simulink model "UNIFIER_3DOFsim"  (R2023b)
settings: Solver=VariableStepAuto  StartTime=0  StopTime=t_sim  RelTol=1e-3
InitFcn:
  | UNIFIER_3DOFsim_init
values from neighbouring files (symbols this model uses):
  b = 20.11467    [UNIFIER_LOAD.m]    (also in UNIFIER_LOAD.mat; UNIFIER_LOAD_ROM.m; UNIFIER_LOAD_ROM.mat)
  c = 1.43676    [UNIFIER_LOAD.m]    (also in UNIFIER_LOAD.mat; UNIFIER_LOAD_ROM.m; UNIFIER_LOAD_ROM.mat)
  DEP_inc = -0.0872664625997    [UNIFIER_LOAD.mat]    (also in UNIFIER_ROMdyn.m = deg2rad(-5); UNIFIER_ROMdyn_script.m = deg2rad(-5); UNIFIER_ROMdyn_v2.m = deg2rad(-5); UNIFIER_ROMgen.m = 0.1)
  dp_DEP =     [UNIFIER_LOAD.mat]    (also in UNIFIER_LOAD_ROM.mat)
  dp_FUSE_FIN =     [UNIFIER_LOAD.mat]
  dp_HTU =     [UNIFIER_LOAD.mat]    (also in UNIFIER_LOAD_ROM.mat)
  dp_VTAIL =     [UNIFIER_LOAD.mat]
  dp_VTAIL_INDUCED =     [UNIFIER_LOAD.mat]
  dp_WING_root =     [UNIFIER_LOAD.mat]
  dp_WING_tip =     [UNIFIER_LOAD.mat]
  dumax = [2.09439510239 2.09439510239 2.09439510239 1.0471975512 2 4 2]    [UNIFIER_LOAD.mat]    (also in UNIFIER_LOAD_ROM.mat = [1.0471975512 1.0471975512 1.0471975512 0.174532925199 2 2 2)
  gr = 9.80665    [UNIFIER_LOAD.mat]    (also in UNIFIER_LOAD_ROM.mat)
  m = 7057    [UNIFIER_LOAD.m]    (also in UNIFIER_LOAD.mat; UNIFIER_LOAD_ROM.m; UNIFIER_LOAD_ROM.mat)
  n_prop = 12    [UNIFIER_LOAD.mat]    (also in UNIFIER_ROMdyn.m; UNIFIER_ROMdyn_script.m; UNIFIER_ROMdyn_v2.m)
  prop_d = 1.6    [UNIFIER_LOAD.mat]    (also in UNIFIER_ROMdyn.m; UNIFIER_ROMdyn_script.m; UNIFIER_ROMdyn_v2.m)
  ROMv1 = ROM    [UNIFIER_3DOFsim_init.m]    (also in UNIFIER_ROMgen_subset.m; UNIFIER_ROMgen_v2_subset.m; UNIFIER_ROMgen_v3_subset.m; UNIFIER_ROMgen_v4_subset.m)
  ROMv2 = ROM    [UNIFIER_3DOFsim_init.m]
  ROMv3 = ROM    [UNIFIER_3DOFsim_init.m]
  S = 29.98388    [UNIFIER_LOAD.m]    (also in UNIFIER_LOAD.mat; UNIFIER_LOAD_ROM.m; UNIFIER_LOAD_ROM.mat)
  U_trim = [ustar(3) ... (first row only)    [UNIFIER_3DOFsim_init.m]
  umax = inf    [UNIFIERLanding.m]    (also in UNIFIER_LOAD.mat = [0.436332312999 0.523598775598 0.523598775598 0.436332312999; UNIFIER_LOAD_ROM.mat = [0.436332312999 0.523598775598 0.349065850399 0.436332312999)
  umin = 0    [UNIFIERLanding.m]    (also in UNIFIER_LOAD.mat = [-0.436332312999 -0.523598775598 -0.523598775598 0 0 -1 -0.5; UNIFIER_LOAD_ROM.mat = [-0.436332312999 -0.523598775598 -0.0872664625997 0 0 -1 0])
  Va = sqrt(u^2+w^2)    [ROMcomp.m]    (also in UNIFIERLanding.m = sqrt(x(:,3).^2+x(:,4).^2); UNIFIERLanding_Dynamics_Internal.m = sqrt(X(:,3).^2+X(:,4).^2); UNIFIERLanding_Main.m = sqrt(solution.X(:,3).^2+solution.X(:,4).^2); UNIFIERLanding_trajopt.m = sqrt(solution.X(:,3).^2+solution.X(:,4).^2))
  vtail_nodes = [dp_VTAIL.Xs_LE;     dp_VTAIL.Ys_LE;     dp_VTAIL.Zs_LE]    [UNIFIER_LOAD.m]    (also in UNIFIER_LOAD.mat = [-16.4894695282 -2.83441376686 -2.73765826225 -16.1370849609)
  wing_nodes = [fliplr(dp_WING_tip.LE_Xs),fliplr(dp_WING_root.LE_Xs),dp_WING_root.LE_Xs,dp_WING_tip.LE_Xs;     fliplr(-dp_WING_tip.LE_Ys),fliplr(-dp_WING_root.LE_Ys),dp_WING_root.LE_Ys,dp_WING_tip.LE_Ys;     fliplr(dp_WING_tip.LE_Zs),fliplr(dp_WING_root.LE_Zs),dp_WING_root.LE_Zs,dp_WING_tip.LE_Zs]    [UNIFIER_LOAD.m]    (also in UNIFIER_LOAD.mat = [-7.70795631409 -9.67500019073 -0.98178178072 -7.66801691055)
  x0 = xstar(1)    [UNIFIERLanding.m]    (also in UNIFIER_3DOFsim_init.m; UNIFIER_dynamics.m = x; UNIFIER_trim.m = [Va_target/100; UNIFIER_trim1.m = [Va_target)
  xstar = [0;        0;        -ze_target;        zstar(1)*100;        0;        zstar(2)*100;        0;        zstar(3);        0;        0;        0;        0]    [UNIFIER_trim.m]    (also in UNIFIER_trim0_res.mat = [0 0 -500 55.1327882403 0 -0.446351795968 0 1.36591182427e-0; UNIFIER_trim1.m = [0;        0;        -ze_target;        zstar(1);        0; ; UNIFIER_trim1_res.mat = [0 0 -1219 72.7310470326 0 1.14230710452 0 0.0157060522827 0; UNIFIER_trimHFM.m = [0;        0;        -runconfig.ze;        zstar(1)*100;    )
  xyz_cg = [-8.09,0,-0.2]    [UNIFIER_LOAD.m]    (also in UNIFIER_LOAD.mat = [-8.09 0 -0.2]; UNIFIER_LOAD_ROM.m; UNIFIER_LOAD_ROM.mat = [-8.09 0 -0.2])
  xyz_cg_12 = [-8.09 0 -0.2 -8.09 0 -0.2 -8.09 0 -0.2 -8.09 0 -0.2 ... (36 elements, 3x12)]    [UNIFIER_LOAD.mat]    (also in UNIFIER_LOAD_ROM.mat)
  xyz_DEP = [ -6.9629998	-6.9210000	-6.8660002	-6.8099999	-6.7540002	-6.6999998	-6.6999998	-6.7540002	-6.8099999	-6.8660002	-6.9210000	-6.9629998 ... (first row only)    [UNIFIER_LOAD.m]    (also in UNIFIER_LOAD.mat = [-6.9629998 -10.05 -0.90899998 -6.921 -8.4499998 -0.792 -6.8; UNIFIER_LOAD_ROM.m; UNIFIER_LOAD_ROM.mat = [-6.9629998 -10.05 -0.90899998 -6.921 -8.4499998 -0.792 -6.8)
  z0 = x(1,2)    [UNIFIERLanding.m]    (also in UNIFIER_3DOFsim_init.m = xstar(3); UNIFIER_trim.m = zstar; UNIFIER_trim1.m = zstar; UNIFIER_trimHFM.m = zstar)
undefined symbols (not defined in the file or in its folder): solution
libraries: simulink_extras x17, sharedutil x5, slpidlib x4, aerolibtransform2 x4, dspindex x2, matrix_library x1, shared6dof x1, aerolibatmos2 x1, simulink x1
(part 1 of 4)
settings Model: Creator=Reggie Johanes  LastModifiedBy=Reggie Johanes
settings DataIOCC: SaveFormat=StructureWithTime
settings OptimizationCC: BlockReduction=off  BufferReuse=off
settings DebuggingCC: AlgebraicLoopMsg=none  ParameterPrecisionLossMsg=none

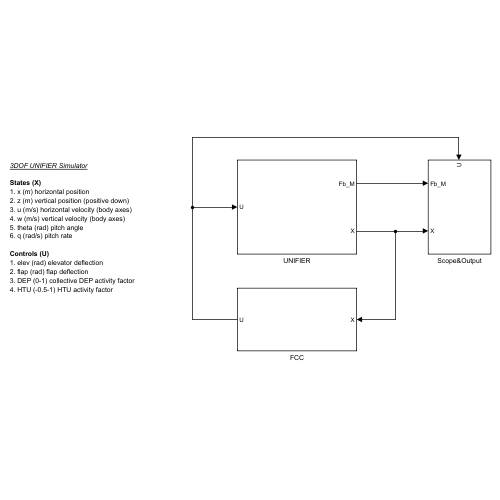
[thumbnail: Simulink's stored preview of the top-level diagram]
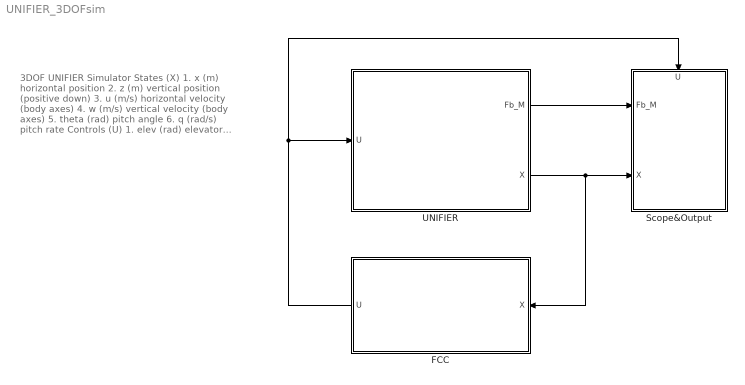
== system UNIFIER_3DOFsim ==
  note: 3DOF UNIFIER Simulator
      |
      | States (X)
      | 1. x (m) horizontal position
      | 2. z (m) vertical position (positive down)
      | 3. u (m/s) horizontal velocity (body axes)
      | 4. w (m/s) vertical velocity (body axes)
      | 5. theta (rad) pitch angle
      | 6. q (rad/s) pitch rate
      |
      | Controls (U)
      | 1. elev (rad) elevator deflection
      | 2. flap (rad) flap deflection
      | 3. DEP (0-1) collective DEP activity factor
      | 4. HTU (-0.5-1) HTU activity factor
  FCC : Subsystem
  Scope&Output : Subsystem
      settings: PortSchema="{\"entries\":[{\"content\":{\"sides\":[{\"content\":{\"connectorIds\":[\"In1\",\"In2\"]},\"type\":\"ConnectorPlacement.EquallySpacedRectSide\",\"uuid\":\"009958d8-f299-4591-8265-ecda8c772736\"},{\"content\":{\"side\":\"RIGHT\"},\"type\":\"ConnectorPlacement.EquallySpacedRectSide\",\"uuid\":\"c33e155a-8705-44ed-ad70-cac76bf4a7ef\"},{\"content\":{\"connectorIds\":[\"In3\"],\"side\":\"TOP\"},\"type\":\"ConnectorPlacement.EquallySpacedRectSide\",\"uuid\":\"edbc7869-8e0d-4a22-bba1-11cba2971ecb\"}]},\"type\":\"ConnectorPlacement.EquallySpacedConnector\",\"uuid\":\"bd1ea077-c17e-402d-9949-f0df00fcfe32\"}],\"packageUris\":[\"http://schema.mathworks.com/mf0/Connector/R2020b\"],\"version\":\"1.0\"}"
  UNIFIER : Subsystem
  wires:
  UNIFIER/2(X) -> FCC/1(X), Scope&Output/2(X)
  FCC/1(U) -> UNIFIER/1(U), Scope&Output/3(U)
  UNIFIER/1(Fb_M) -> Scope&Output/1(Fb_M)

== system UNIFIER_3DOFsim/FCC ==
  X : Inport
  Airspeed Control : Subsystem
      settings: PortSchema="{\"entries\":[{\"content\":{\"sides\":[{\"content\":{\"connectorIds\":[\"In1\",\"In2\"]},\"type\":\"ConnectorPlacement.EquallySpacedRectSide\",\"uuid\":\"a3fb04a8-89c2-4134-89d4-6d6a43062b9b\"},{\"content\":{\"connectorIds\":[\"Out1\"],\"side\":\"RIGHT\"},\"type\":\"ConnectorPlacement.EquallySpacedRectSide\",\"uuid\":\"0d35a5ec-1bbb-45b5-ad25-2bc644cb46ec\"},{\"content\":{\"connectorIds\":[\"Out2\"],\"side\":\"TOP\"},\"type\":\"ConnectorPlacement.EquallySpacedRectSide\",\"uuid\":\"07800402-c5fd-46cf-bb6b-6507cb62190b\"}]},\"type\":\"ConnectorPlacement.EquallySpacedConnector\",\"uuid\":\"0f781fd0-6236-48b8-b612-1777b9bca292\"}],\"packageUris\":[\"http://schema.mathworks.com/mf0/Connector/R2020b\"],\"version\":\"1.0\"}"
  Altitude Control : Subsystem
      settings: PortSchema="{\"entries\":[{\"content\":{\"sides\":[{\"content\":{\"connectorIds\":[\"In1\",\"In2\",\"In3\",\"In4\"]},\"type\":\"ConnectorPlacement.EquallySpacedRectSide\",\"uuid\":\"d6eebd62-3574-4a6b-be51-6258a51c0c28\"},{\"content\":{\"connectorIds\":[\"Out1\"],\"side\":\"RIGHT\"},\"type\":\"ConnectorPlacement.EquallySpacedRectSide\",\"uuid\":\"54870a02-b95d-471b-a2c8-ee83b599c45e\"},{\"content\":{\"side\":\"TOP\"},\"type\":\"ConnectorPlacement.EquallySpacedRectSide\",\"uuid\":\"efdc830e-c8bf-412c-9d86-dbb1e6c1c86b\"},{\"content\":{\"connectorIds\":[\"Out2\"],\"side\":\"BOTTOM\"},\"type\":\"ConnectorPlacement.EquallySpacedRectSide\",\"uuid\":\"beb3ac17-a4c7-4320-a029-baa0478db22b\"}]},\"type\":\"ConnectorPlacement.EquallySpacedConnector\",\"uuid\":\"0f69f6a5-bc47-4551-ad8e-935190b4abb2\"}],\"packageUris\":[\"http://schema.mathworks.com/mf0/Connector/R2020b\"],\"version\":\"1.0\"}"
  Bus Selector : BusSelector  OutputSignals=Va_tas,xe,ze,theta,q
  Constant : Constant  Value=U_trim
  Demux : Demux
  From : From
  Gain : Gain  Commented=through  Gain=0
  Gain1 : Gain  Commented=through  Gain=0
  Goto : Goto
  Mux : Mux
  Sat&RateLimits : Subsystem
  Scopes : Subsystem
      settings: PortSchema="{\"entries\":[{\"content\":{\"sides\":[{\"content\":{},\"type\":\"ConnectorPlacement.EquallySpacedRectSide\",\"uuid\":\"9f44d661-c392-453f-8f32-a438acdd3e9a\"},{\"content\":{\"connectorIds\":[\"In1\",\"In2\",\"In3\",\"In4\"],\"side\":\"RIGHT\"},\"type\":\"ConnectorPlacement.EquallySpacedRectSide\",\"uuid\":\"1fec26d2-6697-4a56-8467-3c40b28ed85c\"},{\"content\":{\"side\":\"TOP\"},\"type\":\"ConnectorPlacement.EquallySpacedRectSide\",\"uuid\":\"ddff103d-3713-4047-b105-bfe64402e206\"}]},\"type\":\"ConnectorPlacement.EquallySpacedConnector\",\"uuid\":\"f87a61e9-3668-4a68-bbee-b53c56c665da\"}],\"packageUris\":[\"http://schema.mathworks.com/mf0/Connector/R2020b\"],\"version\":\"1.0\"}"
  Sum : Sum  Inputs=|++
  Sum1 : Sum  Inputs=|++
  Sum2 : Sum  Inputs=|++
  U : Outport
  wires:
  X/1 -> [C], Bus Selector/1
  Constant/1 -> Demux/1
  Sat&RateLimits/1(U_lim) -> U/1, Scopes/4(U)
  Mux/1 -> Sat&RateLimits/1(U)
  Sum/1 -> Mux/1  "elev"
  Demux/1 -> Sum/2
  Demux/3 -> Sum1/2
  Demux/4 -> Sum2/2
  Sum2/1 -> Mux/4  "HTU"
  Sum1/1 -> Mux/3  "DEP"
  Demux/2 -> Mux/2  "flap"
  Altitude Control/1(elev) -> Gain/1
  Airspeed Control/1(thr) -> Gain1/1
  Bus Selector/1 -> Airspeed Control/1(Va)  "<Va_tas>"
  Bus Selector/2 -> Airspeed Control/2(Xe), Altitude Control/4(Xe)  "<xe>"
  Bus Selector/3 -> Altitude Control/1(Ze)  "<ze>"
  Bus Selector/4 -> Altitude Control/2(theta)  "<theta>"
  Bus Selector/5 -> Altitude Control/3(q)  "<q>"
  Airspeed Control/2(scopeout) -> Goto/1
  Altitude Control/2(scopeout) -> [B]
  From/1 -> Scopes/1(Vactrl)
  [B] -> Scopes/2(altctrl)
  [C] -> Scopes/3(X)
  Gain/1 -> Sum/1
  Gain1/1 -> Sum2/1, Sum1/1

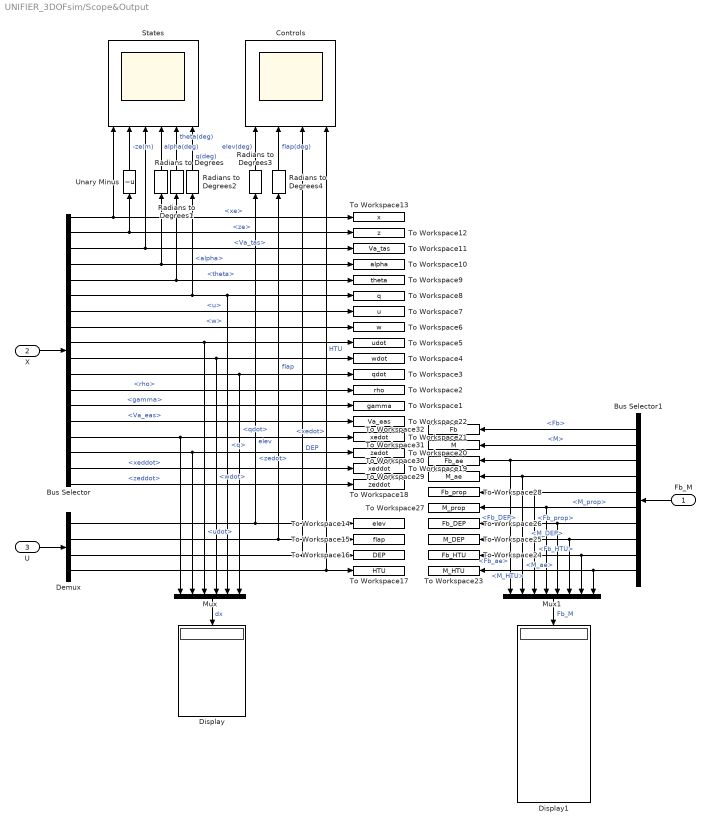
== system UNIFIER_3DOFsim/Scope&Output ==
  Fb_M : Inport
  X : Inport  Port=2
  U : Inport  Port=3
  Bus Selector : BusSelector  OutputSignals=xe,ze,Va_tas,alpha,theta,q,u,w,udot,wdot,qdot,rho,gamma,Va_eas,xedot,zedot,xeddot,zeddot
  Bus Selector1 : BusSelector  OutputSignals=Fb,M,Fb_ae,M_ae,Fb_prop,M_prop,Fb_DEP,M_DEP,Fb_HTU,M_HTU
  Controls : Scope  NumInputPorts=4
  Demux : Demux
  Display : Display
  Display1 : Display
  Mux : Mux  Inputs=6
  Mux1 : Mux  Inputs=8
  Radians to Degrees{,1..4} (5 alike) : simulink_extras/Transformations/Radians to Degrees
  States : Scope  NumInputPorts=6
  To Workspace1 : ToWorkspace  VariableName=gamma  SampleTime=-1
  To Workspace10 : ToWorkspace  VariableName=alpha  SampleTime=-1
  To Workspace11 : ToWorkspace  VariableName=Va_tas  SampleTime=-1
  To Workspace12 : ToWorkspace  VariableName=z  SampleTime=-1
  To Workspace13 : ToWorkspace  VariableName=x  SampleTime=-1
  To Workspace14 : ToWorkspace  VariableName=elev  SampleTime=-1
  To Workspace15 : ToWorkspace  VariableName=flap  SampleTime=-1
  To Workspace16 : ToWorkspace  VariableName=DEP  SampleTime=-1
  To Workspace17 : ToWorkspace  VariableName=HTU  SampleTime=-1
  To Workspace18 : ToWorkspace  VariableName=zeddot  SampleTime=-1
  To Workspace19 : ToWorkspace  VariableName=xeddot  SampleTime=-1
  To Workspace2 : ToWorkspace  VariableName=rho  SampleTime=-1
  To Workspace20 : ToWorkspace  VariableName=zedot  SampleTime=-1
  To Workspace21 : ToWorkspace  VariableName=xedot  SampleTime=-1
  To Workspace22 : ToWorkspace  VariableName=Va_eas  SampleTime=-1
  To Workspace23 : ToWorkspace  VariableName=M_HTU  SampleTime=-1
  To Workspace24 : ToWorkspace  VariableName=Fb_HTU  SampleTime=-1
  To Workspace25 : ToWorkspace  VariableName=M_DEP  SampleTime=-1
  To Workspace26 : ToWorkspace  VariableName=Fb_DEP  SampleTime=-1
  To Workspace27 : ToWorkspace  VariableName=M_prop  SampleTime=-1
  To Workspace28 : ToWorkspace  VariableName=Fb_prop  SampleTime=-1
  To Workspace29 : ToWorkspace  VariableName=M_ae  SampleTime=-1
  To Workspace3 : ToWorkspace  VariableName=qdot  SampleTime=-1
  To Workspace30 : ToWorkspace  VariableName=Fb_ae  SampleTime=-1
  To Workspace31 : ToWorkspace  VariableName=M  SampleTime=-1
  To Workspace32 : ToWorkspace  VariableName=Fb  SampleTime=-1
  To Workspace4 : ToWorkspace  VariableName=wdot  SampleTime=-1
  To Workspace5 : ToWorkspace  VariableName=udot  SampleTime=-1
  To Workspace6 : ToWorkspace  VariableName=w  SampleTime=-1
  To Workspace7 : ToWorkspace  VariableName=u  SampleTime=-1
  To Workspace8 : ToWorkspace  VariableName=q  SampleTime=-1
  To Workspace9 : ToWorkspace  VariableName=theta  SampleTime=-1
  Unary Minus : UnaryMinus
  wires:
  X/1 -> Bus Selector/1
  Bus Selector/1 -> States/1, To Workspace13/1  "<xe>"
  Bus Selector/2 -> Unary Minus/1, To Workspace12/1  "<ze>"
  Bus Selector/3 -> States/3, To Workspace11/1  "<Va_tas>"
  Bus Selector/4 -> Radians to Degrees/1, To Workspace10/1  "<alpha>"
  Bus Selector/5 -> Radians to Degrees1/1, To Workspace9/1  "<theta>"
  Bus Selector/6 -> Radians to Degrees2/1, To Workspace8/1, Mux/5  "<q>"
  Bus Selector/8 -> To Workspace6/1  "<w>"
  Bus Selector/9 -> To Workspace5/1, Mux/3  "<udot>"
  Bus Selector/10 -> To Workspace4/1, Mux/4  "<wdot>"
  Bus Selector/11 -> To Workspace3/1, Mux/6  "<qdot>"
  Bus Selector/12 -> To Workspace2/1  "<rho>"
  Bus Selector/13 -> To Workspace1/1  "<gamma>"
  Bus Selector/7 -> To Workspace7/1  "<u>"
  U/1 -> Demux/1
  Demux/1 -> Radians to Degrees3/1, To Workspace14/1  "elev"
  Demux/2 -> To Workspace15/1, Radians to Degrees4/1  "flap"
  Demux/3 -> To Workspace16/1, Controls/3  "DEP"
  Demux/4 -> To Workspace17/1, Controls/4  "HTU"
  Radians to Degrees/1 -> States/4  "alpha(deg)"
  Radians to Degrees1/1 -> States/5  "theta(deg)"
  Radians to Degrees2/1 -> States/6  "q(deg)"
  Radians to Degrees3/1 -> Controls/1  "elev(deg)"
  Radians to Degrees4/1 -> Controls/2  "flap(deg)"
  Unary Minus/1 -> States/2  "-ze(m)"
  Bus Selector/14 -> To Workspace22/1  "<Va_eas>"
  Bus Selector/15 -> To Workspace21/1, Mux/1  "<xedot>"
  Bus Selector/16 -> To Workspace20/1, Mux/2  "<zedot>"
  Bus Selector/17 -> To Workspace19/1  "<xeddot>"
  Bus Selector/18 -> To Workspace18/1  "<zeddot>"
  Mux/1 -> Display/1  "dx"
  Fb_M/1 -> Bus Selector1/1
  Bus Selector1/3 -> To Workspace30/1, Mux1/1  "<Fb_ae>"
  Bus Selector1/4 -> To Workspace29/1, Mux1/2  "<M_ae>"
  Bus Selector1/5 -> To Workspace28/1, Mux1/3  "<Fb_prop>"
  Bus Selector1/6 -> Mux1/4, To Workspace27/1  "<M_prop>"
  Bus Selector1/7 -> To Workspace26/1, Mux1/5  "<Fb_DEP>"
  Bus Selector1/8 -> To Workspace25/1, Mux1/6  "<M_DEP>"
  Bus Selector1/9 -> To Workspace24/1, Mux1/7  "<Fb_HTU>"
  Bus Selector1/10 -> To Workspace23/1, Mux1/8  "<M_HTU>"
  Mux1/1 -> Display1/1  "Fb_M"
  Bus Selector1/1 -> To Workspace32/1  "<Fb>"
  Bus Selector1/2 -> To Workspace31/1  "<M>"

== system UNIFIER_3DOFsim/UNIFIER ==
  U : Inport
  Aerodynamics : Subsystem
      settings: PortSchema="{\"entries\":[{\"content\":{\"sides\":[{\"content\":{\"connectorIds\":[\"In1\",\"In2\"]},\"type\":\"ConnectorPlacement.EquallySpacedRectSide\",\"uuid\":\"e9d20c59-d6d6-400e-86e2-7a5ce5b582a2\"},{\"content\":{\"connectorIds\":[\"Out1\"],\"side\":\"RIGHT\"},\"type\":\"ConnectorPlacement.EquallySpacedRectSide\",\"uuid\":\"90d146c5-a119-4790-99ca-b691f9272bd7\"},{\"content\":{\"side\":\"TOP\"},\"type\":\"ConnectorPlacement.EquallySpacedRectSide\",\"uuid\":\"d5361e2b-6780-4a80-8d58-884ba2a6b49f\"},{\"content\":{\"connectorIds\":[\"In3\"],\"side\":\"BOTTOM\"},\"type\":\"ConnectorPlacement.EquallySpacedRectSide\",\"uuid\":\"13a1fcba-5f98-490a-a419-e6367cfc3f2c\"}]},\"type\":\"ConnectorPlacement.EquallySpacedConnector\",\"uuid\":\"a6bcc40b-a991-474d-9674-c204f7c17676\"}],\"packageUris\":[\"http://schema.mathworks.com/mf0/Connector/R2020b\"],\"version\":\"1.0\"}"
  EOM&Environment : Subsystem
      settings: PortSchema="{\"entries\":[{\"content\":{\"sides\":[{\"content\":{\"connectorIds\":[\"In1\"]},\"type\":\"ConnectorPlacement.EquallySpacedRectSide\",\"uuid\":\"6160da2b-8552-4ec1-894a-26a5f6c45b78\"},{\"content\":{\"connectorIds\":[\"Out1\",\"Out2\"],\"side\":\"RIGHT\"},\"type\":\"ConnectorPlacement.EquallySpacedRectSide\",\"uuid\":\"7b74025f-6315-4fda-9352-f522b3ee102f\"},{\"content\":{\"side\":\"TOP\"},\"type\":\"ConnectorPlacement.EquallySpacedRectSide\",\"uuid\":\"a0b3834c-0ad6-468f-a161-0f220b7032c2\"},{\"content\":{\"connectorIds\":[\"In2\"],\"side\":\"BOTTOM\"},\"type\":\"ConnectorPlacement.EquallySpacedRectSide\",\"uuid\":\"9d5650a6-6ba4-451c-b870-367e56356c4c\"}]},\"type\":\"ConnectorPlacement.EquallySpacedConnector\",\"uuid\":\"bb7293ac-4d3c-4803-b4ea-767d72af75c5\"}],\"packageUris\":[\"http://schema.mathworks.com/mf0/Connector/R2020b\"],\"version\":\"1.0\"}"
  Propulsion : Subsystem
      settings: PortSchema="{\"entries\":[{\"content\":{\"sides\":[{\"content\":{\"connectorIds\":[\"In1\",\"In2\"]},\"type\":\"ConnectorPlacement.EquallySpacedRectSide\",\"uuid\":\"59a18027-8e03-454d-b478-7172993824c1\"},{\"content\":{\"connectorIds\":[\"Out1\"],\"side\":\"RIGHT\"},\"type\":\"ConnectorPlacement.EquallySpacedRectSide\",\"uuid\":\"f9f30e45-7108-4b05-88e5-0eee1548e389\"},{\"content\":{\"connectorIds\":[\"Out2\"],\"side\":\"TOP\"},\"type\":\"ConnectorPlacement.EquallySpacedRectSide\",\"uuid\":\"8bce0bfc-d093-42df-8b33-22202eb99c5b\"}]},\"type\":\"ConnectorPlacement.EquallySpacedConnector\",\"uuid\":\"2f803787-601f-4bf2-b234-403b5a693950\"}],\"packageUris\":[\"http://schema.mathworks.com/mf0/Connector/R2020b\"],\"version\":\"1.0\"}"
  Fb_M : Outport
  X : Outport  Port=2
  wires:
  Propulsion/1(Fb_M_prop) -> EOM&Environment/2(Fb_M_prop)
  U/1 -> Aerodynamics/2(U), Propulsion/1(U)
  Propulsion/2(J) -> Aerodynamics/3(J)
  Aerodynamics/1(Fb_M_ae) -> EOM&Environment/1(Fb_M_ae)
  EOM&Environment/1(X) -> X/1, Propulsion/2(X), Aerodynamics/1(X)
  EOM&Environment/2(Fb_M) -> Fb_M/1

== system UNIFIER_3DOFsim/FCC/Airspeed Control ==
  Va : Inport
  Xe : Inport  Port=2
  1-D Lookup Table : Lookup_n-D  NumberOfTableDimensions=1  BreakpointsForDimension1=solution.X(:,1)  Table=Va  InternalRulePriority=Speed  RndMeth=Simplest
  1-D Lookup Table1 : Lookup_n-D  Commented=on  NumberOfTableDimensions=1  BreakpointsForDimension1=solution.T  Table=Va  InternalRulePriority=Speed  RndMeth=Simplest
  Bus Creator : BusCreator  Inputs=2
  Clock : Clock  Commented=on
  PID_Va : slpidlib/PID Controller  Controller=PI  Form=Parallel  TimeDomain=Continuous-time  UseExternalTs=off  SampleTime=-1  IntegratorMethod=Forward Euler  FilterMethod=Forward Euler  ControllerParametersSource=internal  P=1.5  I=0.5  UseKiTs=off  D=0.001  N=0  UseFilter=on  TunerSelectOption=Transfer Function Based (PID Tuner App)  InitialConditionSource=internal  InitialConditionForIntegrator=0  InitialConditionForFilter=0  DifferentiatorICPrevScaledInput=0  ExternalReset=none  TrackingMode=off  Kt=1  LimitOutput=off  SatLimitsSource=internal  UpperSaturationLimit=inf  LowerSaturationLimit=-inf  LinearizeAsGain=on  AntiWindupMode=none  Kb=1  LimitIntegrator=off  UpperIntegratorSaturationLimit=inf  LowerIntegratorSaturationLimit=-inf  POutMin=[]  POutMax=[]  IOutMin=[]  IOutMax=[]  DOutMin=[]  DOutMax=[]  NOutMin=[]  NOutMax=[]  SumOutMin=[]  SumOutMax=[]  SaturationOutMin=[]  SaturationOutMax=[]  PParamMin=[]  PParamMax=[]  IParamMin=[]  IParamMax=[]  DParamMin=[]  DParamMax=[]  NParamMin=[]  NParamMax=[]  KbParamMin=[]  KbParamMax=[]  KtParamMin=[]  KtParamMax=[]  KbOutMin=[]  KbOutMax=[]  KtOutMin=[]  KtOutMax=[]  IntegratorOutMin=[]  IntegratorOutMax=[]  FilterOutMin=[]  FilterOutMax=[]  SumI1OutMin=[]  SumI1OutMax=[]  SumI2OutMin=[]  SumI2OutMax=[]  SumI3OutMin=[]  SumI3OutMax=[]  SumI4OutMin=[]  SumI4OutMax=[]  SumDOutMin=[]  SumDOutMax=[]  DifferentiatorOutMin=[]  DifferentiatorOutMax=[]  FilterDiffOutCoefMin=[]  FilterDiffOutCoefMax=[]  ReciprocalOutMin=[]  ReciprocalOutMax=[]  SumDenOutMin=[]  SumDenOutMax=[]  SumNumOutMin=[]  SumNumOutMax=[]  DivideOutMin=[]  DivideOutMax=[]  UdiffTsProdOutMin=[]  UdiffTsProdOutMax=[]  NTsProdOutMin=[]  NTsProdOutMax=[]  UintegralTsProdOutMin=[]  UintegralTsProdOutMax=[]  UngainTsProdOutMin=[]  UngainTsProdOutMax=[]  ClampingZeroOutDataTypeStr=Inherit: Inherit via back propagation  ClampingZeroOutMin=[]  ClampingZeroOutMax=[]  FilterDenConstantOutDataTypeStr=Inherit: Inherit via back propagation  FilterDenConstantOutMin=[]  FilterDenConstantOutMax=[]  PCopyOutDataTypeStr=Inherit: Inherit via back propagation  PCopyOutMin=[]  PCopyOutMax=[]  NCopyOutDataTypeStr=Inherit: Inherit via back propagation  NCopyOutMin=[]  NCopyOutMax=[]  IntegratorContinuousStateAttributes=''  IntegratorStateMustResolveToSignalObject=off  IntegratorRTWStateStorageClass=Auto  FilterContinuousStateAttributes=''  FilterStateMustResolveToSignalObject=off  FilterRTWStateStorageClass=Auto  ParallelPVariant=InternalParameters  IdealPVariant=Disabled  IVariant=InternalParameters  DVariant=Disabled  IntegratorVariant=Continuous  SatVariant=Disabled  AWVariant=Passthrough  PCopyVariant=Disabled  TRVariant=Disabled  FdbkBlocksVariant=Forward  IdealPFdbkVariant=Disabled  SatFdbkVariant=Disabled  DerivativeFilterVariant=Disabled  NVariant=Disabled  NCopyVariant=Disabled_SignalSpec  FilterICVariant=Disabled  IntegratorICVariant=InternalICs  ExternalResetVariant=Disabled  TRSumVariant=Passthrough  SumFdbkVariant=Disabled  SumVariant=Sum_PI  TsampFilterVariant=InternalTs  TsampNgainVariant=Passthrough  TsampIntegralVariant=Disabled_SignalSpec  ExternalSaturationOutDataTypeStr=Inherit: Same as second input
  Sum : Sum  Inputs=|+-
  Sum1 : Sum  Inputs=++|
  Va_ctrl : Scope  NumInputPorts=2
  Va_step : Step  Commented=on  Time=5  Before=72.74  After=72.74  SampleTime=0
  thr : Outport
  scopeout : Outport  Port=2
  wires:
  Va/1 -> Va_ctrl/2, Sum/2
  Sum/1 -> PID_Va/1
  PID_Va/1 -> Bus Creator/2, thr/1  "thr_cmd"
  Xe/1 -> 1-D Lookup Table/1
  1-D Lookup Table/1 -> Sum1/2
  Sum1/1 -> Bus Creator/1, Va_ctrl/1, Sum/1  "Va_ref"
  Bus Creator/1 -> scopeout/1
  Va_step/1 -> Sum1/1
  Clock/1 -> 1-D Lookup Table1/1

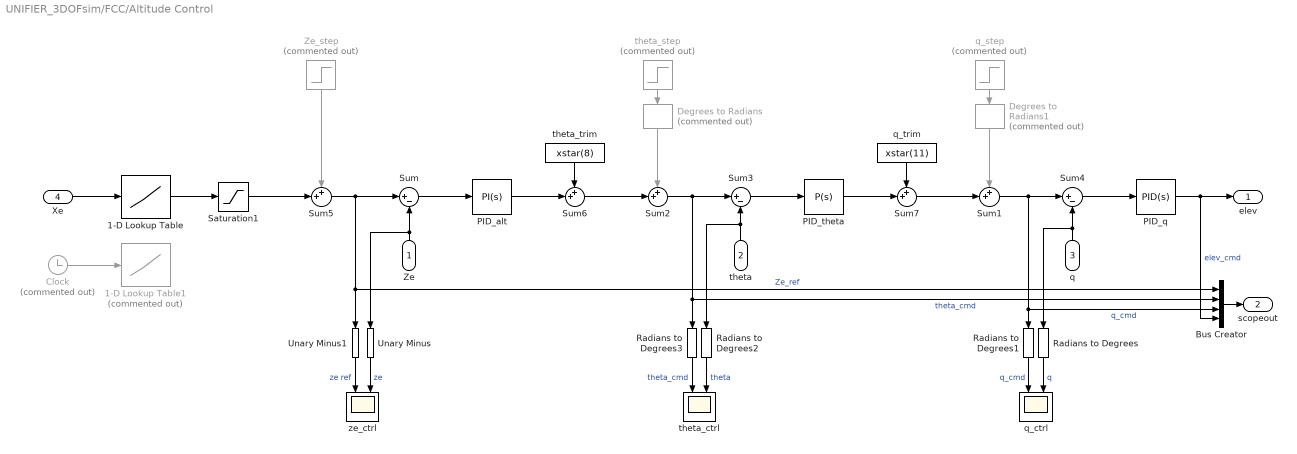
== system UNIFIER_3DOFsim/FCC/Altitude Control ==
  Ze : Inport
  theta : Inport  Port=2
  q : Inport  Port=3
  Xe : Inport  Port=4
  1-D Lookup Table : Lookup_n-D  NumberOfTableDimensions=1  BreakpointsForDimension1=solution.X(:,1)  Table=solution.X(:,2)  InternalRulePriority=Speed  RndMeth=Simplest
  1-D Lookup Table1 : Lookup_n-D  Commented=on  NumberOfTableDimensions=1  BreakpointsForDimension1=solution.T  Table=solution.X(:,2)  InternalRulePriority=Speed  RndMeth=Simplest
  Bus Creator : BusCreator  Inputs=4
  Clock : Clock  Commented=on
  Degrees to Radians : simulink_extras/Transformations/Degrees to Radians  Commented=on
  Degrees to Radians1 : simulink_extras/Transformations/Degrees to Radians  Commented=on
  PID_alt : slpidlib/PID Controller  Controller=PI  Form=Parallel  TimeDomain=Continuous-time  UseExternalTs=off  SampleTime=-1  IntegratorMethod=Forward Euler  FilterMethod=Forward Euler  ControllerParametersSource=internal  P=-0.005  I=-0.001  UseKiTs=off  D=0  N=100  UseFilter=on  TunerSelectOption=Transfer Function Based (PID Tuner App)  InitialConditionSource=internal  InitialConditionForIntegrator=0  InitialConditionForFilter=0  DifferentiatorICPrevScaledInput=0  ExternalReset=none  TrackingMode=off  Kt=1  LimitOutput=off  SatLimitsSource=internal  UpperSaturationLimit=inf  LowerSaturationLimit=-inf  LinearizeAsGain=on  AntiWindupMode=none  Kb=1  LimitIntegrator=off  UpperIntegratorSaturationLimit=inf  LowerIntegratorSaturationLimit=-inf  POutMin=[]  POutMax=[]  IOutMin=[]  IOutMax=[]  DOutMin=[]  DOutMax=[]  NOutMin=[]  NOutMax=[]  SumOutMin=[]  SumOutMax=[]  SaturationOutMin=[]  SaturationOutMax=[]  PParamMin=[]  PParamMax=[]  IParamMin=[]  IParamMax=[]  DParamMin=[]  DParamMax=[]  NParamMin=[]  NParamMax=[]  KbParamMin=[]  KbParamMax=[]  KtParamMin=[]  KtParamMax=[]  KbOutMin=[]  KbOutMax=[]  KtOutMin=[]  KtOutMax=[]  IntegratorOutMin=[]  IntegratorOutMax=[]  FilterOutMin=[]  FilterOutMax=[]  SumI1OutMin=[]  SumI1OutMax=[]  SumI2OutMin=[]  SumI2OutMax=[]  SumI3OutMin=[]  SumI3OutMax=[]  SumI4OutMin=[]  SumI4OutMax=[]  SumDOutMin=[]  SumDOutMax=[]  DifferentiatorOutMin=[]  DifferentiatorOutMax=[]  FilterDiffOutCoefMin=[]  FilterDiffOutCoefMax=[]  ReciprocalOutMin=[]  ReciprocalOutMax=[]  SumDenOutMin=[]  SumDenOutMax=[]  SumNumOutMin=[]  SumNumOutMax=[]  DivideOutMin=[]  DivideOutMax=[]  UdiffTsProdOutMin=[]  UdiffTsProdOutMax=[]  NTsProdOutMin=[]  NTsProdOutMax=[]  UintegralTsProdOutMin=[]  UintegralTsProdOutMax=[]  UngainTsProdOutMin=[]  UngainTsProdOutMax=[]  ClampingZeroOutDataTypeStr=Inherit: Inherit via back propagation  ClampingZeroOutMin=[]  ClampingZeroOutMax=[]  FilterDenConstantOutDataTypeStr=Inherit: Inherit via back propagation  FilterDenConstantOutMin=[]  FilterDenConstantOutMax=[]  PCopyOutDataTypeStr=Inherit: Inherit via back propagation  PCopyOutMin=[]  PCopyOutMax=[]  NCopyOutDataTypeStr=Inherit: Inherit via back propagation  NCopyOutMin=[]  NCopyOutMax=[]  IntegratorContinuousStateAttributes=''  IntegratorStateMustResolveToSignalObject=off  IntegratorRTWStateStorageClass=Auto  FilterContinuousStateAttributes=''  FilterStateMustResolveToSignalObject=off  FilterRTWStateStorageClass=Auto  ParallelPVariant=InternalParameters  IdealPVariant=Disabled  IVariant=InternalParameters  DVariant=Disabled  IntegratorVariant=Continuous  SatVariant=Disabled  AWVariant=Passthrough  PCopyVariant=Disabled  TRVariant=Disabled  FdbkBlocksVariant=Forward  IdealPFdbkVariant=Disabled  SatFdbkVariant=Disabled  DerivativeFilterVariant=Disabled  NVariant=Disabled  NCopyVariant=Disabled_SignalSpec  FilterICVariant=Disabled  IntegratorICVariant=InternalICs  ExternalResetVariant=Disabled  TRSumVariant=Passthrough  SumFdbkVariant=Disabled  SumVariant=Sum_PI  TsampFilterVariant=InternalTs  TsampNgainVariant=Passthrough  TsampIntegralVariant=Disabled_SignalSpec  ExternalSaturationOutDataTypeStr=Inherit: Same as second input
  PID_q : slpidlib/PID Controller  Controller=PID  Form=Parallel  TimeDomain=Continuous-time  UseExternalTs=off  SampleTime=-1  IntegratorMethod=Forward Euler  FilterMethod=Forward Euler  ControllerParametersSource=internal  P=-8.73442191546783  I=-54.0980446276108  UseKiTs=off  D=-0.0407769377294012  N=127.187910258019  UseFilter=on  TunerSelectOption=Transfer Function Based (PID Tuner App)  InitialConditionSource=internal  InitialConditionForIntegrator=0  InitialConditionForFilter=0  DifferentiatorICPrevScaledInput=0  ExternalReset=none  TrackingMode=off  Kt=1  LimitOutput=off  SatLimitsSource=internal  UpperSaturationLimit=inf  LowerSaturationLimit=-inf  LinearizeAsGain=on  AntiWindupMode=none  Kb=1  LimitIntegrator=off  UpperIntegratorSaturationLimit=inf  LowerIntegratorSaturationLimit=-inf  POutMin=[]  POutMax=[]  IOutMin=[]  IOutMax=[]  DOutMin=[]  DOutMax=[]  NOutMin=[]  NOutMax=[]  SumOutMin=[]  SumOutMax=[]  SaturationOutMin=[]  SaturationOutMax=[]  PParamMin=[]  PParamMax=[]  IParamMin=[]  IParamMax=[]  DParamMin=[]  DParamMax=[]  NParamMin=[]  NParamMax=[]  KbParamMin=[]  KbParamMax=[]  KtParamMin=[]  KtParamMax=[]  KbOutMin=[]  KbOutMax=[]  KtOutMin=[]  KtOutMax=[]  IntegratorOutMin=[]  IntegratorOutMax=[]  FilterOutMin=[]  FilterOutMax=[]  SumI1OutMin=[]  SumI1OutMax=[]  SumI2OutMin=[]  SumI2OutMax=[]  SumI3OutMin=[]  SumI3OutMax=[]  SumI4OutMin=[]  SumI4OutMax=[]  SumDOutMin=[]  SumDOutMax=[]  DifferentiatorOutMin=[]  DifferentiatorOutMax=[]  FilterDiffOutCoefMin=[]  FilterDiffOutCoefMax=[]  ReciprocalOutMin=[]  ReciprocalOutMax=[]  SumDenOutMin=[]  SumDenOutMax=[]  SumNumOutMin=[]  SumNumOutMax=[]  DivideOutMin=[]  DivideOutMax=[]  UdiffTsProdOutMin=[]  UdiffTsProdOutMax=[]  NTsProdOutMin=[]  NTsProdOutMax=[]  UintegralTsProdOutMin=[]  UintegralTsProdOutMax=[]  UngainTsProdOutMin=[]  UngainTsProdOutMax=[]  ClampingZeroOutDataTypeStr=Inherit: Inherit via back propagation  ClampingZeroOutMin=[]  ClampingZeroOutMax=[]  FilterDenConstantOutDataTypeStr=Inherit: Inherit via back propagation  FilterDenConstantOutMin=[]  FilterDenConstantOutMax=[]  PCopyOutDataTypeStr=Inherit: Inherit via back propagation  PCopyOutMin=[]  PCopyOutMax=[]  NCopyOutDataTypeStr=Inherit: Inherit via back propagation  NCopyOutMin=[]  NCopyOutMax=[]  IntegratorContinuousStateAttributes=''  IntegratorStateMustResolveToSignalObject=off  IntegratorRTWStateStorageClass=Auto  FilterContinuousStateAttributes=''  FilterStateMustResolveToSignalObject=off  FilterRTWStateStorageClass=Auto  ParallelPVariant=InternalParameters  IdealPVariant=Disabled  IVariant=InternalParameters  DVariant=InternalParameters  IntegratorVariant=Continuous  SatVariant=Disabled  AWVariant=Passthrough  PCopyVariant=Disabled  TRVariant=Disabled  FdbkBlocksVariant=Forward  IdealPFdbkVariant=Disabled  SatFdbkVariant=Disabled  DerivativeFilterVariant=ContFilter  NVariant=InternalParameters  NCopyVariant=Disabled  FilterICVariant=InternalICsFilter  IntegratorICVariant=InternalICs  ExternalResetVariant=Disabled  TRSumVariant=Passthrough  SumFdbkVariant=Disabled  SumVariant=Sum_PID  TsampFilterVariant=InternalTs  TsampNgainVariant=Passthrough  TsampIntegralVariant=Disabled_SignalSpec  ExternalSaturationOutDataTypeStr=Inherit: Same as second input
  PID_theta : slpidlib/PID Controller  Controller=P  Form=Parallel  TimeDomain=Continuous-time  UseExternalTs=off  SampleTime=-1  IntegratorMethod=Forward Euler  FilterMethod=Forward Euler  ControllerParametersSource=internal  P=1.86134542141051  I=7.65203238292703  UseKiTs=off  D=0  N=100  UseFilter=on  TunerSelectOption=Transfer Function Based (PID Tuner App)  InitialConditionSource=internal  InitialConditionForIntegrator=0  InitialConditionForFilter=0  DifferentiatorICPrevScaledInput=0  ExternalReset=none  TrackingMode=off  Kt=1  LimitOutput=off  SatLimitsSource=internal  UpperSaturationLimit=inf  LowerSaturationLimit=-inf  LinearizeAsGain=on  AntiWindupMode=none  Kb=1  LimitIntegrator=off  UpperIntegratorSaturationLimit=inf  LowerIntegratorSaturationLimit=-inf  POutMin=[]  POutMax=[]  IOutMin=[]  IOutMax=[]  DOutMin=[]  DOutMax=[]  NOutMin=[]  NOutMax=[]  SumOutMin=[]  SumOutMax=[]  SaturationOutMin=[]  SaturationOutMax=[]  PParamMin=[]  PParamMax=[]  IParamMin=[]  IParamMax=[]  DParamMin=[]  DParamMax=[]  NParamMin=[]  NParamMax=[]  KbParamMin=[]  KbParamMax=[]  KtParamMin=[]  KtParamMax=[]  KbOutMin=[]  KbOutMax=[]  KtOutMin=[]  KtOutMax=[]  IntegratorOutMin=[]  IntegratorOutMax=[]  FilterOutMin=[]  FilterOutMax=[]  SumI1OutMin=[]  SumI1OutMax=[]  SumI2OutMin=[]  SumI2OutMax=[]  SumI3OutMin=[]  SumI3OutMax=[]  SumI4OutMin=[]  SumI4OutMax=[]  SumDOutMin=[]  SumDOutMax=[]  DifferentiatorOutMin=[]  DifferentiatorOutMax=[]  FilterDiffOutCoefMin=[]  FilterDiffOutCoefMax=[]  ReciprocalOutMin=[]  ReciprocalOutMax=[]  SumDenOutMin=[]  SumDenOutMax=[]  SumNumOutMin=[]  SumNumOutMax=[]  DivideOutMin=[]  DivideOutMax=[]  UdiffTsProdOutMin=[]  UdiffTsProdOutMax=[]  NTsProdOutMin=[]  NTsProdOutMax=[]  UintegralTsProdOutMin=[]  UintegralTsProdOutMax=[]  UngainTsProdOutMin=[]  UngainTsProdOutMax=[]  ClampingZeroOutDataTypeStr=Inherit: Inherit via back propagation  ClampingZeroOutMin=[]  ClampingZeroOutMax=[]  FilterDenConstantOutDataTypeStr=Inherit: Inherit via back propagation  FilterDenConstantOutMin=[]  FilterDenConstantOutMax=[]  PCopyOutDataTypeStr=Inherit: Inherit via back propagation  PCopyOutMin=[]  PCopyOutMax=[]  NCopyOutDataTypeStr=Inherit: Inherit via back propagation  NCopyOutMin=[]  NCopyOutMax=[]  IntegratorContinuousStateAttributes=''  IntegratorStateMustResolveToSignalObject=off  IntegratorRTWStateStorageClass=Auto  FilterContinuousStateAttributes=''  FilterStateMustResolveToSignalObject=off  FilterRTWStateStorageClass=Auto  ParallelPVariant=InternalParameters  IdealPVariant=Disabled  IVariant=Disabled  DVariant=Disabled  IntegratorVariant=Disabled  SatVariant=Disabled  AWVariant=Disabled  PCopyVariant=Disabled  TRVariant=Disabled  FdbkBlocksVariant=Forward  IdealPFdbkVariant=Disabled  SatFdbkVariant=Disabled  DerivativeFilterVariant=Disabled  NVariant=Disabled  NCopyVariant=Disabled_SignalSpec  FilterICVariant=Disabled  IntegratorICVariant=Disabled  ExternalResetVariant=Disabled  TRSumVariant=Passthrough  SumFdbkVariant=Disabled  SumVariant=Passthrough_P  TsampFilterVariant=InternalTs  TsampNgainVariant=Passthrough  TsampIntegralVariant=Disabled_SignalSpec  ExternalSaturationOutDataTypeStr=Inherit: Same as second input
  Radians to Degrees{,1..3} (4 alike) : simulink_extras/Transformations/Radians to Degrees
  Saturation1 : Saturate  UpperLimit=0  LowerLimit=-inf
  Sum : Sum  Inputs=|+-
  Sum{1..2,5..7} (5 alike) : Sum  Inputs=++|
  Sum3 : Sum  Inputs=|+-
  Sum4 : Sum  Inputs=|+-
  Unary Minus : UnaryMinus
  Unary Minus1 : UnaryMinus
  Ze_step : Step  Commented=on  Time=5  Before=-1219  After=-1220  SampleTime=0
  q_ctrl : Scope  NumInputPorts=2
  q_step : Step  Commented=on  Time=5  After=0.1  SampleTime=0
  q_trim : Constant  Value=xstar(11)
  theta_ctrl : Scope  NumInputPorts=2
  theta_step : Step  Commented=on  Time=5  After=0.5  SampleTime=0
  theta_trim : Constant  Value=xstar(8)
  ze_ctrl : Scope  NumInputPorts=2
  elev : Outport
  scopeout : Outport  Port=2
  wires:
  Ze/1 -> Sum/2, Unary Minus/1
  Sum/1 -> PID_alt/1
  q/1 -> Radians to Degrees/1, Sum4/2
  PID_q/1 -> elev/1, Bus Creator/4  "elev_cmd"
  Sum4/1 -> PID_q/1
  Sum3/1 -> PID_theta/1
  theta_step/1 -> Degrees to Radians/1
  q_step/1 -> Degrees to Radians1/1
  Degrees to Radians/1 -> Sum2/1
  Xe/1 -> 1-D Lookup Table/1
  1-D Lookup Table/1 -> Saturation1/1
  Sum5/1 -> Sum/1, Unary Minus1/1, Bus Creator/1  "Ze_ref"
  Sum1/1 -> Bus Creator/3, Radians to Degrees1/1, Sum4/1  "q_cmd"
  Bus Creator/1 -> scopeout/1
  Ze_step/1 -> Sum5/1
  Degrees to Radians1/1 -> Sum1/1
  Saturation1/1 -> Sum5/2
  PID_alt/1 -> Sum6/2
  PID_theta/1 -> Sum7/2
  Clock/1 -> 1-D Lookup Table1/1
  Radians to Degrees/1 -> q_ctrl/2  "q"
  Radians to Degrees1/1 -> q_ctrl/1  "q_cmd"
  Radians to Degrees2/1 -> theta_ctrl/2  "theta"
  theta/1 -> Radians to Degrees2/1, Sum3/2
  Radians to Degrees3/1 -> theta_ctrl/1  "theta_cmd"
  Sum2/1 -> Bus Creator/2, Radians to Degrees3/1, Sum3/1  "theta_cmd"
  Unary Minus/1 -> ze_ctrl/2  "ze"
  Unary Minus1/1 -> ze_ctrl/1  "ze ref"
  Sum6/1 -> Sum2/2
  theta_trim/1 -> Sum6/1
  q_trim/1 -> Sum7/1
  Sum7/1 -> Sum1/2

== system UNIFIER_3DOFsim/FCC/Sat&RateLimits ==
  U : Inport
  DEP : Saturate  UpperLimit=umax(5)  LowerLimit=umin(5)
  Demux : Demux
  HTU : Saturate  UpperLimit=umax(7)  LowerLimit=umin(7)
  Mux : Mux
  Rate Limiter : RateLimiter  RisingSlewLimit=dumax(3)  FallingSlewLimit=-dumax(3)  SampleTimeMode=inherited
  Rate Limiter1 : RateLimiter  RisingSlewLimit=dumax(4)  FallingSlewLimit=-dumax(4)  SampleTimeMode=inherited
  Rate Limiter2 : RateLimiter  RisingSlewLimit=dumax(5)  FallingSlewLimit=-dumax(5)  SampleTimeMode=inherited
  Rate Limiter3 : RateLimiter  RisingSlewLimit=dumax(7)  FallingSlewLimit=-dumax(7)  SampleTimeMode=inherited
  elev : Saturate  UpperLimit=umax(3)  LowerLimit=umin(3)
  flap : Saturate  UpperLimit=umax(4)  LowerLimit=umin(4)
  U_lim : Outport
  wires:
  U/1 -> Demux/1
  Demux/1 -> elev/1
  Demux/2 -> flap/1
  Demux/3 -> DEP/1
  Demux/4 -> HTU/1
  elev/1 -> Rate Limiter/1
  HTU/1 -> Rate Limiter3/1
  DEP/1 -> Rate Limiter2/1
  flap/1 -> Rate Limiter1/1
  Rate Limiter3/1 -> Mux/4
  Rate Limiter2/1 -> Mux/3
  Rate Limiter1/1 -> Mux/2
  Rate Limiter/1 -> Mux/1
  Mux/1 -> U_lim/1

== system UNIFIER_3DOFsim/FCC/Scopes ==
  Vactrl : Inport
  altctrl : Inport  Port=2
  X : Inport  Port=3
  U : Inport  Port=4
  Bus Selector : BusSelector  OutputSignals=ze,theta,q,Va_tas
  Bus Selector1 : BusSelector  OutputSignals=Va_ref,thr_cmd
  Bus Selector2 : BusSelector  OutputSignals=Ze_ref,theta_cmd,q_cmd,elev_cmd
  Demux : Demux
  Radians to Degrees{,1..5} (6 alike) : simulink_extras/Transformations/Radians to Degrees
  Terminator : Terminator
  Unary Minus : UnaryMinus
  Unary Minus1 : UnaryMinus
  Va : Scope  NumInputPorts=2
  elev : Scope  NumInputPorts=2
  q : Scope  NumInputPorts=2
  theta : Scope  NumInputPorts=2
  throttle : Scope  NumInputPorts=3
  ze : Scope  NumInputPorts=2
  wires:
  X/1 -> Bus Selector/1
  Bus Selector/1 -> Unary Minus/1  "<ze>"
  U/1 -> Demux/1
  Bus Selector1/2 -> throttle/3  "<thr_cmd>"
  Bus Selector1/1 -> Va/2  "<Va_ref>"
  Bus Selector/4 -> Va/1  "<Va_tas>"
  Bus Selector/3 -> Radians to Degrees2/1  "<q>"
  Bus Selector/2 -> Radians to Degrees/1  "<theta>"
  Demux/3 -> throttle/1  "DEP"
  Demux/1 -> Radians to Degrees4/1  "elev"
  Demux/2 -> Terminator/1  "flap"
  Demux/4 -> throttle/2  "HTU"
  Bus Selector2/1 -> Unary Minus1/1  "<Ze_ref>"
  Bus Selector2/2 -> Radians to Degrees1/1  "<theta_cmd>"
  Bus Selector2/3 -> Radians to Degrees3/1  "<q_cmd>"
  Bus Selector2/4 -> Radians to Degrees5/1  "<elev_cmd>"
  Unary Minus/1 -> ze/1  "-ze"
  Unary Minus1/1 -> ze/2  "-ze_ref"
  Radians to Degrees/1 -> theta/1
  Radians to Degrees1/1 -> theta/2
  Radians to Degrees2/1 -> q/1
  Radians to Degrees3/1 -> q/2
  Radians to Degrees4/1 -> elev/1
  Radians to Degrees5/1 -> elev/2
  Vactrl/1 -> Bus Selector1/1
  altctrl/1 -> Bus Selector2/1

== system UNIFIER_3DOFsim/UNIFIER/Aerodynamics ==
  note: Choose Model: ROM/HFM
      | (Comment out unused model)
  X : Inport
  U : Inport  Port=2
  J : Inport  Port=3
  Bus Creator : BusCreator  Inputs=2
  HFM : Subsystem
  ROM : Subsystem  Commented=on
  Sum : Sum  Inputs=|++
  Sum1 : Sum  Inputs=|++
  Fb_M_ae : Outport
  wires:
  X/1 -> HFM/1(X), ROM/1(X)
  J/1 -> HFM/3(J), ROM/3(J)
  U/1 -> HFM/2(U), ROM/2(U)
  ROM/1(Fb_ae_ROM) -> Sum/1
  ROM/2(M_ae_ROM) -> Sum1/1
  HFM/1(Fb_ae_HFM) -> Sum/2
  Sum/1 -> Bus Creator/1  "Fb_ae"
  HFM/2(M_ae_HFM) -> Sum1/2
  Sum1/1 -> Bus Creator/2  "M_ae"
  Bus Creator/1 -> Fb_M_ae/1

== system UNIFIER_3DOFsim/UNIFIER/EOM&Environment ==
  note: 3dof block causes algebraic loop error
  Fb_M_ae : Inport
  Fb_M_prop : Inport  Port=2
  3dof (Body Axes) : EOM3DOF  Commented=on  v_ini=Va0  theta_ini=theta0  q_ini=q0  alpha_ini=alpha0  pos_ini=[x0 z0]  mass=m  Iyy=Iyy  g=gr  abi_flag=on
  6dof > 3dof : Subsystem
  AlphaGammaVa : Subsystem
      settings: PortSchema="{\"entries\":[{\"content\":{\"sides\":[{\"content\":{\"connectorIds\":[\"In1\",\"In2\"]},\"type\":\"ConnectorPlacement.EquallySpacedRectSide\",\"uuid\":\"6b7803a5-68fa-4f78-a42f-9a647b75d667\"},{\"content\":{\"connectorIds\":[\"Out1\",\"Out2\",\"Out3\",\"Out4\"],\"side\":\"RIGHT\"},\"type\":\"ConnectorPlacement.EquallySpacedRectSide\",\"uuid\":\"bfe4f380-ec73-417b-97da-72e8837cfba4\"},{\"content\":{\"side\":\"TOP\"},\"type\":\"ConnectorPlacement.EquallySpacedRectSide\",\"uuid\":\"f083671d-0339-4409-a840-6a02be60591e\"},{\"content\":{\"connectorIds\":[\"In3\"],\"side\":\"BOTTOM\"},\"type\":\"ConnectorPlacement.EquallySpacedRectSide\",\"uuid\":\"731baf55-932e-49c8-8708-e52aed641f05\"}]},\"type\":\"ConnectorPlacement.EquallySpacedConnector\",\"uuid\":\"35f468a0-0fbf-4dea-af77-7a5aa13ba4e6\"}],\"packageUris\":[\"http://schema.mathworks.com/mf0/Connector/R2020b\"],\"version\":\"1.0\"}"
  Atmosphere : aerolibatmos2/ISA Atmosphere Model  useExtended=off  action=Warning  custom=off  viscosityOut=off  g=9.80665  gamma=1.4  R=287.0531  L=0.0065  h_trop=11000  h_strat=20000  rho0=1.225  P0=101325  T0=288.15  h0=0
  Bus Creator : BusCreator  Inputs=10
  Bus Creator1 : BusCreator  Inputs=18
  Bus Selector : BusSelector  OutputSignals=Fb_ae,M_ae
  Bus Selector1 : BusSelector  OutputSignals=Fb_prop,M_prop,Fb_DEP,M_DEP,Fb_HTU,M_HTU
  Demux{1..3,5..6} (5 alike) : Demux  Outputs=2
  Demux4 : Demux  Commented=on  Outputs=2
  Sum : Sum  Inputs=++|
  Sum1 : Sum  Inputs=|++
  Terminator : Terminator
  Terminator1 : Terminator
  Terminator2 : Terminator
  Unary Minus : UnaryMinus
  X : Outport
  Fb_M : Outport  Port=2
  wires:
  6dof > 3dof/4(xe ze) -> Demux1/1
  6dof > 3dof/5(u w) -> AlphaGammaVa/1(uw), Demux2/1
  6dof > 3dof/6(udot wdot) -> Demux3/1
  Demux3/2 -> Bus Creator1/5  "wdot"
  Demux3/1 -> Bus Creator1/6  "udot"
  Demux2/2 -> Bus Creator1/7  "w"
  Demux2/1 -> Bus Creator1/8  "u"
  Demux1/2 -> Bus Creator1/9, Unary Minus/1  "ze"
  Bus Creator1/1 -> X/1
  Demux1/1 -> Bus Creator1/10  "xe"
  6dof > 3dof/3(qdot) -> Bus Creator1/11  "qdot"
  6dof > 3dof/2(q) -> Bus Creator1/12  "q"
  6dof > 3dof/1(theta) -> Bus Creator1/13, AlphaGammaVa/2(theta)  "theta"
  Atmosphere/4 -> Bus Creator1/14, AlphaGammaVa/3(rho)  "rho"
  Atmosphere/1 -> Terminator/1
  Atmosphere/2 -> Terminator1/1
  Atmosphere/3 -> Terminator2/1
  AlphaGammaVa/3(Va_tas) -> Bus Creator1/16  "Va_tas"
  AlphaGammaVa/1(alpha) -> Bus Creator1/18  "alpha"
  AlphaGammaVa/2(gamma) -> Bus Creator1/17  "gamma"
  AlphaGammaVa/4(Va_eas) -> Bus Creator1/15  "Va_eas"
  Demux4/1 -> 3dof (Body Axes)/1
  Demux4/2 -> 3dof (Body Axes)/2
  6dof > 3dof/8(xeddot zeddot) -> Demux6/1
  6dof > 3dof/7(xedot zedot) -> Demux5/1
  Demux5/2 -> Bus Creator1/3  "zedot"
  Demux5/1 -> Bus Creator1/4  "xedot"
  Demux6/1 -> Bus Creator1/2  "xeddot"
  Demux6/2 -> Bus Creator1/1  "zeddot"
  Fb_M_ae/1 -> Bus Selector/1
  Fb_M_prop/1 -> Bus Selector1/1
  Sum/1 -> 6dof > 3dof/2(M_3DOF), Bus Creator/10  "M"
  Bus Selector1/2 -> Sum/2, Bus Creator/4  "<M_prop>"
  Sum1/1 -> 6dof > 3dof/1(Fb_3DOF), Bus Creator/9  "Fb"
  Bus Selector/1 -> Sum1/1, Bus Creator/1  "<Fb_ae>"
  Bus Selector/2 -> Sum/1, Bus Creator/2  "<M_ae>"
  Bus Selector1/1 -> Sum1/2, Bus Creator/3  "<Fb_prop>"
  Bus Selector1/3 -> Bus Creator/5  "<Fb_DEP>"
  Bus Selector1/4 -> Bus Creator/6  "<M_DEP>"
  Bus Selector1/5 -> Bus Creator/7  "<Fb_HTU>"
  Bus Selector1/6 -> Bus Creator/8  "<M_HTU>"
  Bus Creator/1 -> Fb_M/1
  Unary Minus/1 -> Atmosphere/1

== system UNIFIER_3DOFsim/UNIFIER/Propulsion ==
  note: HTU subsystem copied from UNIFIER OBM
  note: DEP subsystem reconstructed from UNIFIER OBM with minor changes for 3DOF calculations
  U : Inport
  X : Inport  Port=2
  Bus Creator : BusCreator  Inputs=6
  Bus Selector : BusSelector  OutputSignals=u,rho,Va_eas
  DEP_3DOF : Subsystem
  Demux : Demux  Outputs=2
  HTU : Subsystem
  Selector : Selector  InputPortWidth=4  IndexOptions=Index vector (dialog)  Indices=[3 4]  OutputSizes=1
  Sum : Sum  Inputs=|++
  Sum1 : Sum  Inputs=|++
  Terminator : Terminator
  Terminator1 : Terminator
  Fb_M_prop : Outport
  J : Outport  Port=2
  wires:
  U/1 -> Selector/1
  X/1 -> Bus Selector/1
  Selector/1 -> Demux/1
  DEP_3DOF/1(DEP_J) -> J/1
  DEP_3DOF/2(Fb_DEP) -> Bus Creator/1, Sum/1  "Fb_DEP"
  DEP_3DOF/3(M_DEP) -> Bus Creator/2, Sum1/1  "M_DEP"
  HTU/1(Fb_HTU) -> Bus Creator/3, Sum/2  "Fb_HTU"
  Demux/1 -> DEP_3DOF/3(DEP_col)  "DEP"
  Demux/2 -> HTU/2(HTU)  "HTU"
  Bus Selector/1 -> DEP_3DOF/1(u)  "<u>"
  Bus Selector/2 -> DEP_3DOF/2(rho)  "<rho>"
  Bus Selector/3 -> HTU/1(Va_eas)  "<Va_eas>"
  Sum/1 -> Bus Creator/5  "Fb_prop"
  Sum1/1 -> Bus Creator/6  "M_prop"
  HTU/2(M_HTU) -> Bus Creator/4, Sum1/2  "M_HTU"
  Bus Creator/1 -> Fb_M_prop/1
  DEP_3DOF/4(P_DEP (W)) -> Terminator/1
  HTU/3(P_HTU (W)) -> Terminator1/1

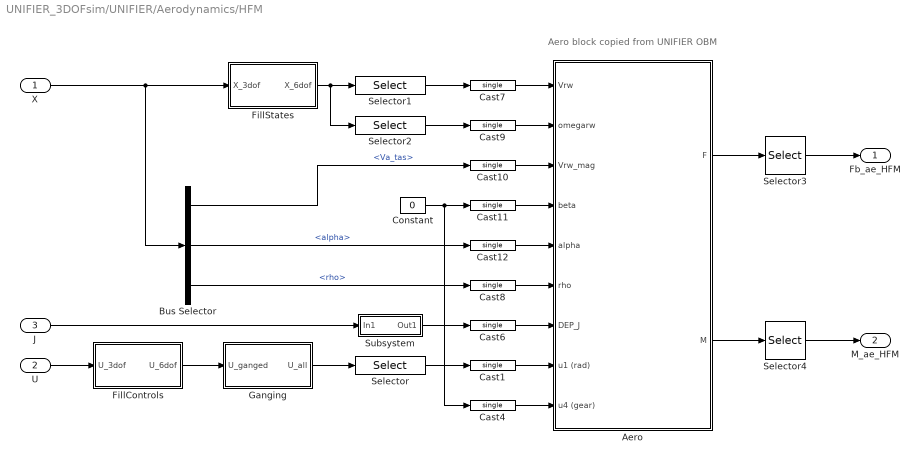
== system UNIFIER_3DOFsim/UNIFIER/Aerodynamics/HFM ==
  note: Aero block copied from UNIFIER OBM
  X : Inport
  U : Inport  Port=2
  J : Inport  Port=3
  Aero : Subsystem
  Bus Selector : BusSelector  OutputSignals=Va_tas,alpha,rho
  Cast{1,4,6..12} (9 alike) : DataTypeConversion  OutDataTypeStr=single  SaturateOnIntegerOverflow=off  RndMeth=Floor
  Constant : Constant  Value=0
  FillControls : Subsystem
  FillStates : Subsystem
  Ganging : Subsystem
  Selector : Selector  InputPortWidth=20  IndexOptions=Index vector (dialog)  Indices=[1:6]  OutputSizes=1
  Selector1 : Selector  InputPortWidth=12  IndexOptions=Index vector (dialog)  Indices=[4 5 6]  OutputSizes=1
  Selector2 : Selector  InputPortWidth=12  IndexOptions=Index vector (dialog)  Indices=[10 11 12]  OutputSizes=1
  Selector3 : Selector  InputPortWidth=3  IndexOptions=Index vector (dialog)  Indices=[1 3]  OutputSizes=1
  Selector4 : Selector  InputPortWidth=3  IndexOptions=Index vector (dialog)  Indices=[2]  OutputSizes=1
  Subsystem : Subsystem
  Fb_ae_HFM : Outport
  M_ae_HFM : Outport  Port=2
  wires:
  Cast9/1 -> Aero/2(omegarw)
  Cast6/1 -> Aero/7(DEP_J)
  Cast11/1 -> Aero/4(beta)
  Cast8/1 -> Aero/6(rho)
  Cast12/1 -> Aero/5(alpha)
  Cast7/1 -> Aero/1(Vrw)
  Cast4/1 -> Aero/9(u4 (gear))
  Cast10/1 -> Aero/3(Vrw_mag)
  Constant/1 -> Cast4/1, Cast11/1
  U/1 -> FillControls/1(U_3dof)
  FillControls/1(U_6dof) -> Ganging/1(U_ganged)
  Ganging/1(U_all) -> Selector/1
  Selector/1 -> Cast1/1
  J/1 -> Subsystem/1(In1)
  X/1 -> FillStates/1(X_3dof), Bus Selector/1
  FillStates/1(X_6dof) -> Selector2/1, Selector1/1
  Selector1/1 -> Cast7/1
  Selector2/1 -> Cast9/1
  Bus Selector/1 -> Cast10/1  "<Va_tas>"
  Bus Selector/3 -> Cast8/1  "<rho>"
  Bus Selector/2 -> Cast12/1  "<alpha>"
  Aero/1(F) -> Selector3/1
  Aero/2(M) -> Selector4/1
  Selector4/1 -> M_ae_HFM/1
  Selector3/1 -> Fb_ae_HFM/1
  Subsystem/1(Out1) -> Cast6/1
  Cast1/1 -> Aero/8(u1 (rad))

== system UNIFIER_3DOFsim/UNIFIER/Aerodynamics/ROM ==
  note: Choose ROM version
      | (Comment out unused versions)
  X : Inport
  U : Inport  Port=2
  J : Inport  Port=3
  Bus Selector : BusSelector  OutputSignals=rho,Va_tas,alpha
  Demux : Demux  Outputs=2
  Gain : Gain  Gain=S
  Gain3 : Gain  Gain=c
  Mux : Mux  Inputs=2
  Product : Product
  Product1 : Product
  Product2 : Product
  ROMv1 : Subsystem
  ROMv2 : Subsystem  Commented=on
  ROMv3 : Subsystem  Commented=on
  Selector : Selector  InputPortWidth=4  IndexOptions=Index vector (dialog)  Indices=[1 2]  OutputSizes=1
  Sum{,1..5} (6 alike) : Sum  Inputs=|++
  calcDynamicPresure : Subsystem
  wind2body : Subsystem
      settings: PortSchema="{\"entries\":[{\"content\":{\"sides\":[{\"content\":{\"connectorIds\":[\"In1\",\"In2\"]},\"type\":\"ConnectorPlacement.EquallySpacedRectSide\",\"uuid\":\"73ecfe4e-53d5-4462-8335-f55aec1625ff\"},{\"content\":{\"connectorIds\":[\"Out1\",\"Out2\"],\"side\":\"RIGHT\"},\"type\":\"ConnectorPlacement.EquallySpacedRectSide\",\"uuid\":\"7be1f14d-b15c-40ee-aca1-1f1bd6d80755\"},{\"content\":{\"connectorIds\":[\"In3\"],\"side\":\"TOP\"},\"type\":\"ConnectorPlacement.EquallySpacedRectSide\",\"uuid\":\"d054d701-1aa9-4d4a-aa52-eaa956b9829f\"}]},\"type\":\"ConnectorPlacement.EquallySpacedConnector\",\"uuid\":\"4b2709be-c0b0-4386-8242-ab405c7af8db\"}],\"packageUris\":[\"http://schema.mathworks.com/mf0/Connector/R2020b\"],\"version\":\"1.0\"}"
  Fb_ae_ROM : Outport
  M_ae_ROM : Outport  Port=2
  wires:
  ROMv2/1(CL) -> Sum3/1
  Demux/1 -> ROMv3/2(elev), ROMv1/2(elev), ROMv2/2(elev)  "elev"
  Bus Selector/3 -> wind2body/3(alpha), ROMv3/1(alpha), ROMv2/1(alpha), ROMv1/1(alpha)  "<alpha>"
  Gain/1 -> Product/1, Gain3/1, Product1/1
  Demux/2 -> ROMv1/3(flap), ROMv2/3(flap)  "flap"
  Bus Selector/2 -> calcDynamicPresure/2(Va)  "<Va_tas>"
  ROMv1/1(CL) -> Sum/1
  Product2/1 -> M_ae_ROM/1  "M"
  Selector/1 -> Demux/1
  Sum/1 -> Product/2
  ROMv2/2(CD) -> Sum4/1
  Bus Selector/1 -> calcDynamicPresure/1(rho)  "<rho>"
  Product1/1 -> wind2body/2(D)  "D"
  ROMv3/3(CM) -> Sum5/2
  Product/1 -> wind2body/1(L)  "L"
  calcDynamicPresure/1(Q) -> Gain/1
  ROMv2/3(CM) -> Sum5/1
  ROMv1/2(CD) -> Sum1/1
  ROMv3/1(CL) -> Sum3/2
  Sum2/1 -> Product2/1
  Sum1/1 -> Product1/2
  Sum5/1 -> Sum2/2
  wind2body/1(Fb_ae_x) -> Mux/1
  ROMv3/2(CD) -> Sum4/2
  Gain3/1 -> Product2/2
  Sum4/1 -> Sum1/2
  ROMv1/3(CM) -> Sum2/1
  X/1 -> Bus Selector/1
  Sum3/1 -> Sum/2
  wind2body/2(Fb_ae_z) -> Mux/2
  U/1 -> Selector/1
  J/1 -> ROMv1/4(J)
  Mux/1 -> Fb_ae_ROM/1
